simulink model "linear_system_angelo"  (R2016a)
settings: Solver=VariableStepAuto  SolverMode=SingleTasking  StartTime=0.0  StopTime=10.0  RelTol=1e-3
values from neighbouring files (symbols this model uses):
  e = 1/(13640000*0.9989)    (= 7.33945169599e-08)    [entrega3_polos_zeros.m]
  f = d/0.9989    (= 1.34528232943e-10)    [entrega3_polos_zeros.m]
  g = (79/43100)*e    (= 1.34528232943e-10)    [entrega3_polos_zeros.m]
  i = (1/4310000000)+h    (= 2.32265144557e-10)    [entrega3_polos_zeros.m]    (also in plota_graficos.m = i+1)
undefined symbols (not defined in the file or in its folder): fx, fy, mz
settings Model: Creator=diogo  LastModifiedBy=diogo
settings DataIOCC: ReturnWorkspaceOutputs=on
settings DebuggingCC: SFUnexpectedBacktrackingDiag=error  SFNoUnconditionalDefaultTransitionDiag=error
settings SFSimCC: SimUseLocalCustomCode=on
settings RTWCC: RTWUseLocalCustomCode=on
settings GRTTargetCC: TargetLangStandard=C99 (ISO)
settings ConfigComp: CovMetricSettings=dwe  CovHtmlReporting=off  CovSaveCumulativeToWorkspaceVar=off  CovSaveSingleToWorkspaceVar=off  CovExternalEMLEnable=on

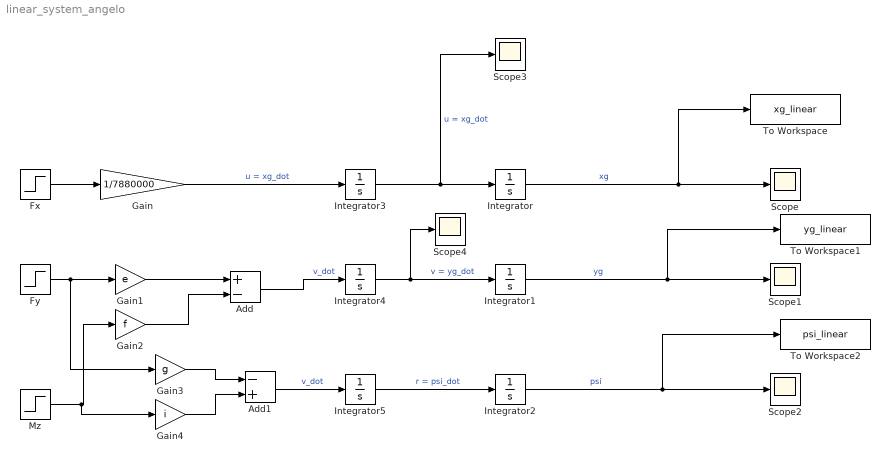
== system linear_system_angelo ==
  Add : Sum  Inputs=+-
  Add1 : Sum  Inputs=-+
  Fx : Step  Time=0  After=fx  SampleTime=0
  Fy : Step  Time=0  After=fy  SampleTime=0
  Gain : Gain  Gain=1/7880000
  Gain1 : Gain  Gain=e
  Gain2 : Gain  Gain=f
  Gain3 : Gain  Gain=g
  Gain4 : Gain  Gain=i
  Integrator{,1..5} (6 alike) : Integrator
  Mz : Step  Time=0  After=mz  SampleTime=0
  Scope{,1..4} (5 alike) : Scope
  To Workspace : ToWorkspace  VariableName=xg_linear  SaveFormat=Timeseries  SampleTime=-1
  To Workspace1 : ToWorkspace  VariableName=yg_linear  SaveFormat=Timeseries  SampleTime=-1
  To Workspace2 : ToWorkspace  VariableName=psi_linear  SaveFormat=Timeseries  SampleTime=-1
  wires:
  Integrator/1 -> To Workspace/1, Scope/1  "xg"
  Integrator3/1 -> Scope3/1, Integrator/1  "u = xg_dot"
  Integrator1/1 -> To Workspace1/1, Scope1/1  "yg"
  Integrator2/1 -> To Workspace2/1, Scope2/1  "psi"
  Integrator5/1 -> Integrator2/1  "r = psi_dot"
  Integrator4/1 -> Scope4/1, Integrator1/1  "v = yg_dot"
  Fx/1 -> Gain/1
  Gain/1 -> Integrator3/1  "u = xg_dot"
  Fy/1 -> Gain3/1, Gain1/1
  Gain1/1 -> Add/1
  Mz/1 -> Gain4/1, Gain2/1
  Gain2/1 -> Add/2
  Add/1 -> Integrator4/1  "v_dot"
  Gain3/1 -> Add1/1
  Gain4/1 -> Add1/2
  Add1/1 -> Integrator5/1  "v_dot"
